simulink model "PMSG"  (R2020a)
settings: Solver=VariableStepAuto  StartTime=0.0  StopTime=20  RelTol=1e-3
PreLoadFcn:
  | Start_Turbine
InitFcn:
  | Start_Turbine
values from neighbouring files (symbols this model uses):
  id0 = 1.5    [Start_Turbine.m]
  iq0 = 2000    [Start_Turbine.m]
  sampling = 0.01    [Start_Turbine.m]
  w0 = 2    [Start_Turbine.m]
undefined symbols (not defined in the file or in its folder): sigbuilder_block
settings Model: Creator=nccre  LastModifiedBy=nccre

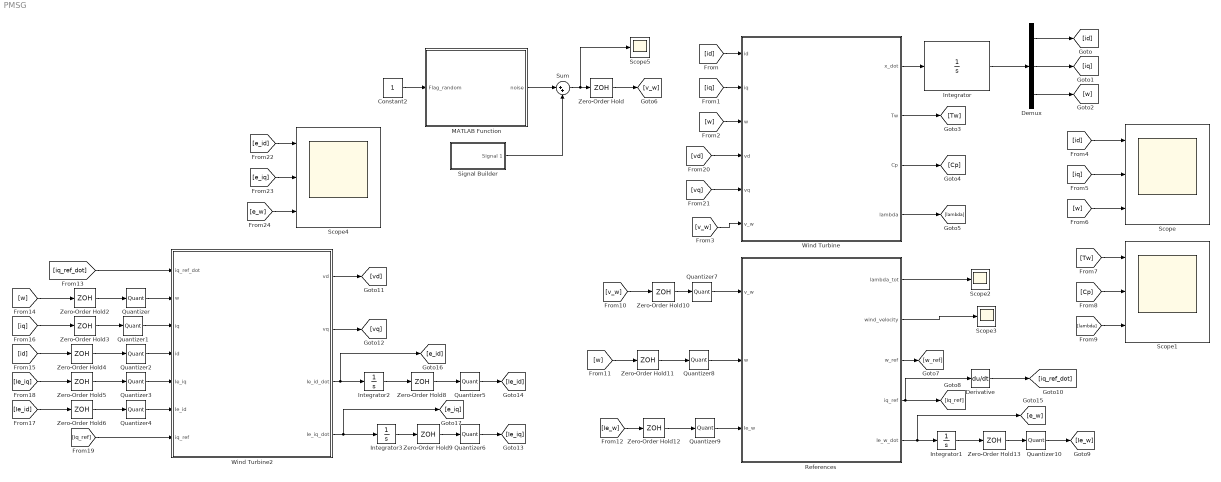
== system PMSG ==
  Constant2 : Constant
  Demux : Demux  Outputs=3
  Derivative : Derivative
  Integrator : Integrator  InitialCondition=[id0;iq0;w0]
  Integrator1 : Integrator
  Integrator2 : Integrator
  Integrator3 : Integrator
  MATLAB Function : MATLAB Function  TreatAsAtomicUnit=on
  Quantizer{,1..10} (11 alike) : Quantizer  QuantizationInterval=quantization_error
  References : MATLAB Function  TreatAsAtomicUnit=on
  Scope : Scope  NumInputPorts=3
  Scope1 : Scope  NumInputPorts=3
  Scope2 : Scope
  Scope3 : Scope
  Scope4 : Scope  NumInputPorts=3
  Scope5 : Scope
  Signal Builder : Subsystem  Tag=STV Subsys  LoadFcn=sigbuilder_block('load');  StartFcn=sigbuilder_block('start');  StopFcn=sigbuilder_block('stop');  ClipboardFcn=sigbuilder_block('clipboard');  mask(Sigbuilder block){tuvar=[0:10]}
      mask help: Simulink:masks:SigbuilderBlock_MD
      mask init:
      | if ~strcmp(get_param(bdroot(gcbh),'SimulationStatus'),'stopped') tuvar = sigbuilder_block('maskInit'); end
      settings: CopyFcn=sigbuilder_block('copy');  DeleteFcn=sigbuilder_block('delete');  ModelCloseFcn=sigbuilder_block('modelClose');  PreSaveFcn=sigbuilder_block('preSave');  PauseFcn=sigbuilder_block('pause');  ContinueFcn=sigbuilder_block('continue');  NameChangeFcn=sigbuilder_block('namechange');  OpenFcn=sigbuilder_block('open',[5.4 33 1141.2 514.8 ]);  CloseFcn=sigbuilder_block('close');
      mask Display: plot(0, 0, 100, 100,[2, 2, 32, 32, 2], [68, 8, 8, 68, 68],[32, 2], [38, 38], [32, 19, 2],[53, 60, 44], [32, 17, 17, 2],[16, 16, 31, 31]);txt = getActiveGroup(gcbh);text(2, 100, txt,'verticalAlignment', 'top');
  Sum : Sum  Inputs=|++
  Wind Turbine : MATLAB Function  TreatAsAtomicUnit=on
  Wind Turbine2 : MATLAB Function  TreatAsAtomicUnit=on
  Zero-Order Hold{,2..6,8..13} (12 alike) : ZeroOrderHold  SampleTime=sampling
  wires:
  Wind Turbine/1(x_dot) -> Integrator/1
  Integrator/1 -> Demux/1
  Demux/3 -> [w]
  Demux/2 -> [iq]
  Demux/1 -> [id]
  Wind Turbine/2(Tw) -> [Tw]
  Wind Turbine/3(Cp) -> [Cp]
  Wind Turbine/4(lambda) -> [lambda]
  [iq] -> Wind Turbine/2(iq)
  [id] -> Wind Turbine/1(id)
  [w] -> Wind Turbine/3(w)
  Constant2/1 -> MATLAB Function/1(Flag_random)
  MATLAB Function/1(noise) -> Sum/1
  Signal Builder/1(Signal 1) -> Sum/2
  Sum/1 -> Scope5/1, Zero-Order Hold/1
  [v_w] -> Wind Turbine/6(v_w)
  [w] -> Scope/3
  [iq] -> Scope/2
  [id] -> Scope/1
  [Tw] -> Scope1/1
  [Cp] -> Scope1/2
  [lambda] -> Scope1/3
  [v_w] -> Zero-Order Hold10/1
  [w] -> Zero-Order Hold11/1
  References/1(lambda_tot) -> Scope2/1
  References/2(wind_velocity) -> Scope3/1
  References/4(iq_ref) -> Derivative/1, [iq_ref]
  References/5(Ie_w_dot) -> [e_w], Integrator1/1
  Integrator1/1 -> Zero-Order Hold13/1
  [Ie_w] -> Zero-Order Hold12/1
  References/3(w_ref) -> [w_ref]
  Derivative/1 -> [iq_ref_dot]
  [w] -> Zero-Order Hold2/1
  [iq] -> Zero-Order Hold3/1
  [id] -> Zero-Order Hold4/1
  Wind Turbine2/3(Ie_id_dot) -> [e_id], Integrator2/1
  Wind Turbine2/4(Ie_iq_dot) -> [e_iq], Integrator3/1
  Wind Turbine2/1(vd) -> [vd]
  Wind Turbine2/2(vq) -> [vq]
  Integrator2/1 -> Zero-Order Hold8/1
  Integrator3/1 -> Zero-Order Hold9/1
  [Ie_id] -> Zero-Order Hold6/1
  [Ie_iq] -> Zero-Order Hold5/1
  [vd] -> Wind Turbine/4(vd)
  [vq] -> Wind Turbine/5(vq)
  [e_id] -> Scope4/1
  [e_w] -> Scope4/3
  [e_iq] -> Scope4/2
  Zero-Order Hold/1 -> [v_w]
  [iq_ref_dot] -> Wind Turbine2/1(iq_ref_dot)
  Zero-Order Hold2/1 -> Quantizer/1
  Zero-Order Hold3/1 -> Quantizer1/1
  Zero-Order Hold4/1 -> Quantizer2/1
  Zero-Order Hold5/1 -> Quantizer3/1
  Zero-Order Hold6/1 -> Quantizer4/1
  [iq_ref] -> Wind Turbine2/7(iq_ref)
  Zero-Order Hold8/1 -> Quantizer5/1
  Zero-Order Hold9/1 -> Quantizer6/1
  Zero-Order Hold10/1 -> Quantizer7/1
  Zero-Order Hold11/1 -> Quantizer8/1
  Zero-Order Hold13/1 -> Quantizer10/1
  Zero-Order Hold12/1 -> Quantizer9/1
  Quantizer/1 -> Wind Turbine2/2(w)
  Quantizer1/1 -> Wind Turbine2/3(iq)
  Quantizer2/1 -> Wind Turbine2/4(id)
  Quantizer3/1 -> Wind Turbine2/5(Ie_iq)
  Quantizer4/1 -> Wind Turbine2/6(Ie_id)
  Quantizer5/1 -> [Ie_id]
  Quantizer6/1 -> [Ie_iq]
  Quantizer7/1 -> References/1(v_w)
  Quantizer8/1 -> References/2(w)
  Quantizer9/1 -> References/3(Ie_w)
  Quantizer10/1 -> [Ie_w]

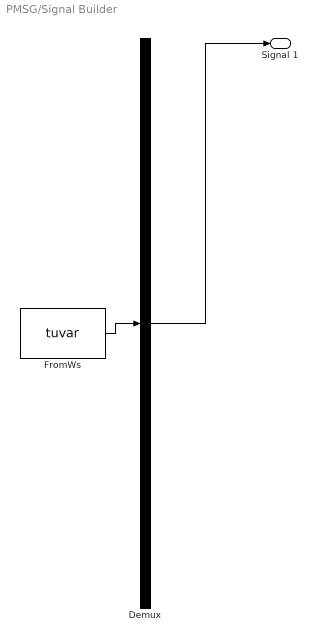
== system PMSG/Signal Builder ==
  Demux : Demux  Tag=STV Demux  Outputs=1
      settings: DisplayOption=none
  FromWs : FromWorkspace  Tag=STV FromWs  VariableName=tuvar
      SigBuilderData=|
      | common.afterFinalStr = 'Extrapolate'
      | common.sampleTime = 0
      | dataSet.timeRange = [0 10]
      | dataSet.name = 'Group 1'
      | sbobj.Groups.Name = 'Group 1'
      | sbobj.Groups.Signals.Name = 'Signal 1'
      | sbobj.Groups.Signals.XData = [0 1.9 2.9 8 8.2 10]
      | sbobj.Groups.Signals.YData = [7 7 9.4 9.4 9 9]
  Signal 1 : Outport  Tag=STV Outport
  wires:
  Demux/1 -> Signal 1/1
  FromWs/1 -> Demux/1

== matlab function PMSG/MATLAB Function ==
  data: Flag_random input; noise output
function noise  = wind_noise(Flag_random)
noise=Flag_random*0.005*randi([-10,10]);
end

== matlab function PMSG/Wind Turbine ==
  data: id input; x_dot output; iq input; w input; vd input; vq input; v_w input; Tw output; Cp output; lambda output
function [x_dot,Tw,Cp,lambda] = model(id,iq,w,vd,vq,v_w)
%#eml
eml.extrinsic('evalin');

% Loading parameters from workspace
% Initialization

R=0;
Rs=0;
L=0;
phim=0;
p=0;
J=0;
f=0;
km=0;
c1=0;
c2=0;
c3=0;
c4=0;
c5=0;
c6=0;
rho=0;

% Take the parameters from the workspace

R=evalin('base','R');
Rs=evalin('base','Rs');
L=evalin('base','L');
phim=evalin('base','phim');
p=evalin('base','p');
J=evalin('base','J');
f=evalin('base','f');
km=evalin('base','km');
c1=evalin('base','c1');
c2=evalin('base','c2');
c3=evalin('base','c3');
c4=evalin('base','c4');
c5=evalin('base','c5');
c6=evalin('base','c6');
rho=evalin('base','rho');

% Definition of the model

lambda=(w*R)/v_w;
C_p=c1*(c2*(1/lambda-c3)-c4)*exp(-c5*(1/lambda-c3))+c6*lambda;
if C_p>0
    Cp=C_p;
else
    Cp=0;
end

T_w=(rho*pi*R^5*Cp*w^2)/(2*lambda^3); %T_w=kw*w^2
if T_w>0
    Tw=T_w;
else
    Tw=0;
end


id_dot=-(Rs/L)*id+p*w*iq+(vd/L);
iq_dot=-(Rs/L)*iq-p*w*id-(p*phim*w)/L+(vq/L);
w_dot=-(km/J)*iq-(f/J)*w+(Tw/J);

x_dot=[id_dot;iq_dot;w_dot];
end

== matlab function PMSG/References ==
  data: v_w input; w input; Ie_w input; lambda_tot output; wind_velocity output; w_ref output; iq_ref output; Ie_w_dot output
function [lambda_tot,wind_velocity,w_ref,iq_ref,Ie_w_dot] = reference_generator(v_w,w,Ie_w)
%#eml
eml.extrinsic('evalin');

% Loading parameters from workspace
% Initialization



R=0;
Rs=0;
L=0;
phim=0;
p=0;
J=0;
f=0;
km=0;
c1=0;
c2=0;
c3=0;
c4=0;
c5=0;
c6=0;
rho=0;
lambda_max=0;

% Take the parameters from the workspace

R=evalin('base','R');
Rs=evalin('base','Rs');
L=evalin('base','L');
phim=evalin('base','phim');
p=evalin('base','p');
J=evalin('base','J');
f=evalin('base','f');
km=evalin('base','km');
c1=evalin('base','c1');
c2=evalin('base','c2');
c3=evalin('base','c3');
c4=evalin('base','c4');
c5=evalin('base','c5');
c6=evalin('base','c6');
rho=evalin('base','rho');
lambda_max=evalin('base','lambda_max');

% Real tip speed ratio
lambda=(w*R)/v_w;
C_p=c1*(c2*(1/lambda-c3)-c4)*exp(-c5*(1/lambda-c3))+c6*lambda;
if C_p>0
    Cp=C_p;
else
    Cp=0;
end

% Real torque due to the wind

kw=(rho*pi*R^5*Cp)/(2*lambda^3);
T_w=kw*w^2;
if T_w>0
    Tw=T_w;
else
    Tw=0;
end

% Estimation of the wind velocity

v_wh0=7.5; % Initial value of the estimated wind velocity
lambda_h=(w*R)/v_wh0; % Initial value of the estimated tip speed ratio
C_ph=c1*(c2*(1/lambda_h-c3)-c4)*exp(-c5*(1/lambda_h-c3))+c6*lambda_h;
if C_ph>0
    Cph=C_ph;
else
    Cph=0;
end

kw0=(rho*pi*R^5*Cph)/(2*lambda_h^3);
T_w0=kw0*w^2;
if T_w0>0
    Tw0=T_w0;
else
    Tw0=0;
end
a1=c1*(-c2*c3/lambda_h-c2*(-c3*lambda_h+1)/lambda_h^2)*exp(-c5*(-c3*lambda_h+1)/lambda_h+c4)+c1*(c2*(-c3*lambda_h+1)/lambda_h-c4)*(c5*c3/lambda_h+c5*(-c3*lambda_h+1)/lambda_h^2)*exp(-c5*(-c3*lambda_h+1)/lambda_h+c4)+c6;
a2=3*(c1*(c2*(-c3*lambda_h+1)/lambda_h-c4)*exp(-c5*(-c3*lambda_h+1)/lambda_h+c4)+c6*lambda_h);
DCp=a1/lambda_h^3-a2/lambda_h^4;


Pm=kw*w^3;

f_lambda=Pm-kw0*w^3;
df_lambda=-(rho*pi*R^5*w^3*DCp)/2;

N=109;
% Newton-Raphson method
for i=1:N
    lambda_h=lambda_h-f_lambda/df_lambda;
end

C_ph=c1*(c2*(1/lambda_h-c3)-c4)*exp(-c5*(1/lambda_h-c3))+c6*lambda_h;
if C_ph>0
    Cph=C_ph;
else
    Cph=0;
end
kw0=(rho*pi*R^5*Cph)/(2*lambda_h^3);
T_w0=kw0*w^2;
if T_w0>0
    Tw0=T_w0;
else
    Tw0=0;
end
lambda_tot=[lambda;lambda_h];
v_wh=w*R/lambda_h;
wind_velocity=[v_w;v_wh];

w_ref=lambda_max*v_wh/R;

kp2=30;
ki2=2*kp2;

e_w=w-w_ref;

Ie_w_dot=e_w;

iq_ref=J/km*(-(f/J)*w+(Tw0/J)+kp2*e_w+ki2*Ie_w);
end

== matlab function PMSG/Wind Turbine2 ==
  data: iq_ref_dot input; vd output; vq output; w input; iq input; id input; Ie_iq input; Ie_id input; iq_ref input; Ie_id_dot output; Ie_iq_dot output
function [vd,vq,Ie_id_dot,Ie_iq_dot] = controller(iq_ref_dot,w,iq,id,Ie_iq,Ie_id,iq_ref)
%#eml
eml.extrinsic('evalin');

% Loading parameters from workspace
% Initialization



R=0;
Rs=0;
L=0;
phim=0;
p=0;
J=0;
f=0;
km=0;
c1=0;
c2=0;
c3=0;
c4=0;
c5=0;
c6=0;
rho=0;
lambda_max=0;

% Take the parameters from the workspace

R=evalin('base','R');
Rs=evalin('base','Rs');
L=evalin('base','L');
phim=evalin('base','phim');
p=evalin('base','p');
J=evalin('base','J');
f=evalin('base','f');
km=evalin('base','km');
c1=evalin('base','c1');
c2=evalin('base','c2');
c3=evalin('base','c3');
c4=evalin('base','c4');
c5=evalin('base','c5');
c6=evalin('base','c6');
rho=evalin('base','rho');
lambda_max=evalin('base','lambda_max');

% Definition of the controller
id_ref=0;
e_id=id-id_ref;
Ie_id_dot=e_id;

kp1=30;
ki1=2*kp1;
vd=L*((Rs/L)*id-p*w*iq-kp1*e_id-ki1*Ie_id);

e_iq=iq-iq_ref;
Ie_iq_dot=e_iq;

kp3=30;
ki3=2*kp3;

vq=L*((Rs/L)*iq+p*w*id+(p*phim*w)/L-kp3*e_iq-ki3*Ie_iq+iq_ref_dot);


end
